simulink model "ES200A_CurrMeas"  (R2013b)
settings: Solver=FixedStepDiscrete  SolverMode=SingleTasking  StartTime=0.0  StopTime=1  FixedStep=0.000125  RelTol=1e-3
undefined symbols (not defined in the file): ARCHGLBPRM_2PI_ULS_F32, CurrMeasEolGainMax, CurrMeasEolGainMin, CurrMeasEolGainNrOfSample, CurrMeasEolGainNumer, CurrMeasEolMaxMotVel, CurrMeasEolOffsHiBrdgVltgMin, CurrMeasEolOffsHiCmuOffs, CurrMeasEolOffsLoCmuOffs, CurrMeasEolOffsMax, CurrMeasEolOffsMin, CurrMeasEolOffsNrOfSample, CurrMeasEolTranCntrThd, CurrMeasMinRqrdPhaOnTi, CurrMeasMotAgCompuDly, CurrMeasMotCurrAdcVlyWrmIninMax, CurrMeasMotCurrAdcVlyWrmIninMin, CurrMeasNtc0x05DFailStep, CurrMeasNtc0x05DPassStep, CurrMeasNtc0x06DFailStep, CurrMeasNtc0x06DPassStep, DEGREES30_MOTRAD_F32, DIFOFFSRNGCHKMAX_VOLT_F32, ELECGLBPRM_IVTRCNT_CNT_U08, ELECGLBPRM_STRTUPSTCURRMEASWRMININTESTSTRT_CNT_U08, FLTINJ_CURRMEAS_MOTCURRCORRDA, FLTINJ_CURRMEAS_MOTCURRCORRDD, FLTINJ_CURRMEAS_TESTOK, MAXCURRCORRD_AMPR_F32, PhaABCMeasdOutOfRng, PhaDEFMeasOutOfRng, SysGlbPrmMotPoleCnt
libraries: simulink x10, FixdToFloat x1
(part 4 of 7)

== system ES200A_CurrMeas/CurrMeas/CurrMeasInit1/If Action Subsystem1 ==
  Action Port : ActionPort  ActionType=else
  Constant{,1..5} (6 alike) : Constant  Value=0  OutDataTypeStr=single
  MotCurrOffsDeltaA : Outport
  MotCurrOffsDeltaB : Outport  Port=2
  MotCurrOffsDeltaC : Outport  Port=3
  MotCurrOffsDeltaD : Outport  Port=4
  MotCurrOffsDeltaE : Outport  Port=5
  MotCurrOffsDeltaF : Outport  Port=6
  wires:
  Constant2/1 -> MotCurrOffsDeltaC/1  "MotCurrOffDeltaC"
  Constant1/1 -> MotCurrOffsDeltaB/1  "MotCurrOffDeltaB"
  Constant/1 -> MotCurrOffsDeltaA/1  "MotCurrOffDeltaA"
  Constant3/1 -> MotCurrOffsDeltaD/1
  Constant4/1 -> MotCurrOffsDeltaE/1
  Constant5/1 -> MotCurrOffsDeltaF/1

== system ES200A_CurrMeas/CurrMeas/CurrMeasOffsReadReq/CopyRight2 ==

== system ES200A_CurrMeas/CurrMeas/CurrMeasOffsWrReq/CopyRight2 ==

== system ES200A_CurrMeas/CurrMeas/CurrMeasOffsWrReq/IF ==
  CurrMeasEolOffsHiBrdgVltg_ArgIn : Inport  RequirementInfo={} %GIDa_812a1a2f_8d9b_493f_8d38_cf559d2e2313  OutDataTypeStr=single
  CurrMeasMotCurrOffsDifA_ArgIn : Inport  RequirementInfo={} %GIDa_620df217_6d23_4379_b697_2438223fdb1e  Port=2  OutDataTypeStr=single
  CurrMeasMotCurrOffsLoAvrgA_ArgIn : Inport  RequirementInfo={} %GIDa_fbdbb2e3_d8ba_4172_b27f_3be627a5f176  Port=3  OutDataTypeStr=single
  CurrMeasMotCurrOffsLoAvrgB_ArgIn : Inport  RequirementInfo={} %GIDa_4342fbfc_d634_403b_9b29_d8803beea53e  Port=4  OutDataTypeStr=single
  CurrMeasMotCurrOffsLoAvrgC_ArgIn : Inport  RequirementInfo={} %GIDa_1155a904_daa1_442b_9b3a_76183cfeb8de  Port=5  OutDataTypeStr=single
  CurrMeasMotCurrOffsLoAvrgD_ArgIn : Inport  RequirementInfo={} %GIDa_b5928048_b518_475c_bd85_7d449910b834  Port=6  OutDataTypeStr=single
  CurrMeasMotCurrOffsLoAvrgE_ArgIn : Inport  RequirementInfo={} %GIDa_2f4f2a2a_6567_449e_882d_b458829ff196  Port=7  OutDataTypeStr=single
  CurrMeasMotCurrOffsLoAvrgF_ArgIn : Inport  RequirementInfo={} %GIDa_a7fe6648_99b2_41ba_8ec9_da3c20c2e7af  Port=8  OutDataTypeStr=single
  CurrMeasMotCurrOffsDifB_ArgIn : Inport  RequirementInfo={} %GIDa_17cf677d_9485_4eb6_bf0d_5d95365246ca  Port=9  OutDataTypeStr=single
  CurrMeasMotCurrOffsDifC_ArgIn : Inport  RequirementInfo={} %GIDa_8d171d0b_2ff9_462a_9ae6_84a29f9d80d8  Port=10  OutDataTypeStr=single
  CurrMeasMotCurrOffsDifD_ArgIn : Inport  RequirementInfo={} %GIDa_84414505_75c9_4dd9_ba80_d7374193ac56  Port=11  OutDataTypeStr=single
  CurrMeasMotCurrOffsDifE_ArgIn : Inport  RequirementInfo={} %GIDa_d54e2248_e490_46ca_9d40_ef0ba9a5a858  Port=12  OutDataTypeStr=single
  CurrMeasMotCurrOffsDifF_ArgIn : Inport  RequirementInfo={} %GIDa_15e5f242_fd24_4678_b9cf_ed0d82bfd499  Port=13  OutDataTypeStr=single
  Action Port : ActionPort  ActionType=then
  Constant14 : Constant  OutDataTypeStr=single
  CurrMeasEolOffsCalSet : DataStoreWrite  RequirementInfo={'linktype_rmi_doors' '000089bc (/ESG Group/FDD Module Requirements/EA4 Specific/ES200A_CurrMeas)' '#ES200A_280' 'true' 'REQ: ES200A_280' '' } %GIDa_65bd6eae_4bc4_46b4_a91f_58c4237add93  DataStoreName=CurrMeasEolOffsCalSet  DataStoreElements=CurrMeasEolOffsCalSet.CurrMeasEolOffsHiBrdgVltg#CurrMeasEolOffsCalSet.CurrMeasMotCurrEolOffsDifA#CurrMeasEolOffsCalSet.CurrMeasMotCurrEolOffsDifB#CurrMeasEolOffsCalSet.CurrMeasMotCurrEolOffsDifC#CurrMeasEolOffsCalSet.CurrMeasMotCurrEolOffsDifD#CurrMeasEolOffsCalSet.CurrMeasMotCurrEolOffsDifE#CurrMeasEolOffsCalSet.CurrMeasMotCurrEolOffsDifF#CurrMeasEolOffsCalSet.CurrMeasMotCurrOffsLoAvrgA#CurrMeasEolOffsCalSet.CurrMeasMotCurrOffsLoAvrgB#CurrMeasEolOffsCalSet.CurrMeasMotCurrOffsLoAvrgC#CurrMeasEolOffsCalSet.CurrMeasMotCurrOffsLoAvrgD#CurrMeasEolOffsCalSet.CurrMeasMotCurrOffsLoAvrgE#CurrMeasEolOffsCalSet.CurrMeasMotCurrOffsLoAvrgF
  CurrMeasEolOffsCalSet_SetRamBlockStatus : Subsystem  RequirementInfo={'linktype_rmi_doors' '000089bc (/ESG Group/FDD Module Requirements/EA4 Specific/ES200A_CurrMeas)' '#ES200A_280' 'true' 'REQ: ES200A_280' '' } %GIDa_fdbbe63c_7b7e_430e_a45c_f1a2eec3b0d3  TreatAsAtomicUnit=on
  Positive Response : Constant  Value=0
  CurrMeasOffsWrReqSts : Outport  RequirementInfo={} %GIDa_d6bd7840_4b1f_429e_aa0e_09addb50176a
  wires:
  CurrMeasMotCurrOffsDifB_ArgIn/1 -> CurrMeasEolOffsCalSet/3
  CurrMeasMotCurrOffsDifA_ArgIn/1 -> CurrMeasEolOffsCalSet/2
  CurrMeasMotCurrOffsLoAvrgC_ArgIn/1 -> CurrMeasEolOffsCalSet/10
  CurrMeasMotCurrOffsLoAvrgD_ArgIn/1 -> CurrMeasEolOffsCalSet/11
  CurrMeasMotCurrOffsLoAvrgF_ArgIn/1 -> CurrMeasEolOffsCalSet/13
  CurrMeasMotCurrOffsDifF_ArgIn/1 -> CurrMeasEolOffsCalSet/7
  CurrMeasMotCurrOffsDifC_ArgIn/1 -> CurrMeasEolOffsCalSet/4
  CurrMeasMotCurrOffsDifE_ArgIn/1 -> CurrMeasEolOffsCalSet/6
  CurrMeasMotCurrOffsLoAvrgB_ArgIn/1 -> CurrMeasEolOffsCalSet/9
  CurrMeasMotCurrOffsDifD_ArgIn/1 -> CurrMeasEolOffsCalSet/5
  CurrMeasMotCurrOffsLoAvrgA_ArgIn/1 -> CurrMeasEolOffsCalSet/8
  CurrMeasMotCurrOffsLoAvrgE_ArgIn/1 -> CurrMeasEolOffsCalSet/12
  Constant14/1 -> CurrMeasEolOffsCalSet_SetRamBlockStatus/1("BlockChanged ")
  CurrMeasEolOffsHiBrdgVltg_ArgIn/1 -> CurrMeasEolOffsCalSet/1
  Positive Response/1 -> CurrMeasOffsWrReqSts/1

== system ES200A_CurrMeas/CurrMeas/CurrMeasOffsWrReq/else  ==
  Action Port : ActionPort  ActionType=else
  Negative Response : Constant
  CurrMeasOffsWrReqSts : Outport  RequirementInfo={} %GIDa_bbade129_568d_4f6a_aeaa_1c5484c89fdb
  wires:
  Negative Response/1 -> CurrMeasOffsWrReqSts/1

== system ES200A_CurrMeas/CurrMeas/CurrMeasPer1/CopyRight2 ==

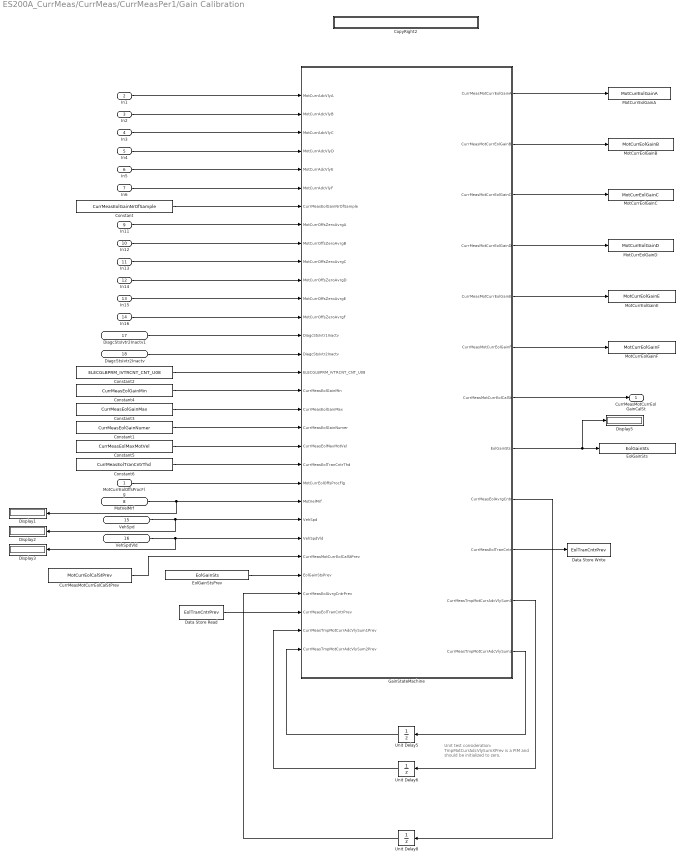
== system ES200A_CurrMeas/CurrMeas/CurrMeasPer1/Gain Calibration ==
  note: Unit test consideration:
      | TmpMotCurrAdcVlySumXPrev is a PIM
      | and should be initialized to zero.
  MotCurrEolOffsProcFlg : Inport
  In1 : Inport  Port=2
  In2 : Inport  Port=3
  In3 : Inport  Port=4
  In4 : Inport  Port=5
  In5 : Inport  Port=6
  In6 : Inport  Port=7
  MotVelMrf : Inport  RequirementInfo={} %GIDa_a7b78662_7cf0_48ed_9f87_08134d024c78  Port=8  OutDataTypeStr=single
  In11 : Inport  Port=9
  In12 : Inport  Port=10
  In13 : Inport  Port=11
  In14 : Inport  Port=12
  In15 : Inport  Port=13
  In16 : Inport  Port=14
  VehSpd : Inport  RequirementInfo={} %GIDa_c841d099_fc23_4afc_9dd2_bf4d1285ca82  Port=15
  VehSpdVld : Inport  RequirementInfo={} %GIDa_a5c49bc6_dd19_4849_b83d_4c3bf1157af9  Port=16  OutDataTypeStr=single
  DiagcStsIvtr2Inactv1 : Inport  RequirementInfo={} %GIDa_8700043e_90fa_4116_85b4_a3555476b354  Port=17
  DiagcStsIvtr2Inactv : Inport  RequirementInfo={} %GIDa_425966d8_d289_4e11_9dbb_57044454bfa8  Port=18
  Constant : Constant  Value=CurrMeasEolGainNrOfSample
  Constant1 : Constant  Value=CurrMeasEolGainNumer
  Constant2 : Constant  Value=ELECGLBPRM_IVTRCNT_CNT_U08  OutDataTypeStr=uint8
  Constant3 : Constant  Value=CurrMeasEolGainMax
  Constant4 : Constant  Value=CurrMeasEolGainMin
  Constant5 : Constant  Value=CurrMeasEolMaxMotVel
  Constant6 : Constant  Value=CurrMeasEolTranCntrThd
  CopyRight2 : Subsystem  Description=|  mask(Copyright Information){none=on}
      | Copyright info block.                                               
      |                                                                     
      | Place copyright information at the top of every subsystem in design.
      mask prompts: none "No parameters"
      mask help: Place copyright information at the top of every subsystem in design.
      mask Display:
      | NxtrConf = 'Nexteer Confidential';
      | 
      | sys = bdroot; %handle for the current model ("system")
      | first = get_param(sys,'Created');
      | first = first(end-3:end);  %year is last four digits
      | 
      | last = get_param(sys,'LastModifiedDate');
      | if isempty(last)
      |     last = datestr(now,'yyyy');
      | else
      |     last = last(end-3:end);
      | end
      | 
      | if strcmp(first,last)
      |     fprintf('%s -- Copyright %s Nexteer',NxtrConf,first)
      | else
      |     fprintf('%s -- %s%s- %s Nexteer',NxtrConf,char(169),first,last)
      | end
  CurrMeasMotCurrEolCalStPrev : DataStoreRead  DataStoreName=MotCurrEolCalStPrev  DataStoreElements=MotCurrEolCalStPrev
  Data Store Read : DataStoreRead  DataStoreName=EolTranCntrPrev
  Data Store Write : DataStoreWrite  DataStoreName=EolTranCntrPrev
  Display{1..3,5} (4 alike) : Display
  EolGainSts : DataStoreWrite  DataStoreName=EolGainSts
  EolGainStsPrev : DataStoreRead  DataStoreName=EolGainSts  DataStoreElements=EolGainSts
  GainStateMachine : Stateflow chart  RequirementInfo={'linktype_rmi_doors' '000089bc (/ESG Group/FDD Module Requirements/EA4 Specific/ES200A_CurrMeas)' '#ES200A_174' 'true' 'REQ: ES200A_174' '' } %GIDa_289e43b1_cfe4_41ba_9e49_3210dfe736ba  TreatAsAtomicUnit=on
  MotCurrEolGainA : DataStoreWrite  RequirementInfo={} %GIDa_13893fc7_c204_439f_bffc_cfe8ef3246c0  DataStoreName=MotCurrEolGainA
  MotCurrEolGainB : DataStoreWrite  RequirementInfo={} %GIDa_bd072951_11b3_473d_b14d_56675fe847ea  DataStoreName=MotCurrEolGainB
  MotCurrEolGainC : DataStoreWrite  RequirementInfo={} %GIDa_85f7aa39_8d03_4989_9937_397e0bbdc0c3  DataStoreName=MotCurrEolGainC
  MotCurrEolGainD : DataStoreWrite  RequirementInfo={} %GIDa_b5965ed2_4a8c_4234_8376_930d7494d8ae  DataStoreName=MotCurrEolGainD
  MotCurrEolGainE : DataStoreWrite  RequirementInfo={} %GIDa_5641d146_2eac_4d29_ad9c_8f8105bea573  DataStoreName=MotCurrEolGainE
  MotCurrEolGainF : DataStoreWrite  RequirementInfo={} %GIDa_25d2bb4a_a4ab_4b72_9cc3_33d4fd2a8c29  DataStoreName=MotCurrEolGainF
  Unit Delay5 : UnitDelay  SampleTime=-1  StateName=TmpMotCurrAdcVlySum2Prev  StateMustResolveToSignalObject=on
      settings: AttributesFormatString=|
      | State Variable:
      | %<StateName>
  Unit Delay6 : UnitDelay  SampleTime=-1  StateName=TmpMotCurrAdcVlySum1Prev  StateMustResolveToSignalObject=on
      settings: AttributesFormatString=|
      | State Variable:
      | %<StateName>
  Unit Delay8 : UnitDelay  SampleTime=-1  StateName=GainEolAvrgCntrPrev  StateMustResolveToSignalObject=on
      settings: AttributesFormatString=|
      | State Variable:
      | %<StateName>
  CurrMeasMotCurrEolGainCalSt : Outport  OutDataTypeStr=Enum: MotCurrEolCalSt2
  wires:
  GainStateMachine/1(CurrMeasMotCurrEolGainA) -> MotCurrEolGainA/1
  GainStateMachine/2(CurrMeasMotCurrEolGainB) -> MotCurrEolGainB/1
  GainStateMachine/3(CurrMeasMotCurrEolGainC) -> MotCurrEolGainC/1
  GainStateMachine/5(CurrMeasMotCurrEolGainE) -> MotCurrEolGainE/1
  GainStateMachine/6(CurrMeasMotCurrEolGainF) -> MotCurrEolGainF/1
  GainStateMachine/4(CurrMeasMotCurrEolGainD) -> MotCurrEolGainD/1
  GainStateMachine/8(EolGainSts) -> Display5/1, EolGainSts/1
  GainStateMachine/7(CurrMeasMotCurrEolCalSt) -> CurrMeasMotCurrEolGainCalSt/1
  In14/1 -> GainStateMachine/11(MotCurrOffsZeroAvrgD)
  In15/1 -> GainStateMachine/12(MotCurrOffsZeroAvrgE)
  In16/1 -> GainStateMachine/13(MotCurrOffsZeroAvrgF)
  In11/1 -> GainStateMachine/8(MotCurrOffsZeroAvrgA)
  In12/1 -> GainStateMachine/9(MotCurrOffsZeroAvrgB)
  In13/1 -> GainStateMachine/10(MotCurrOffsZeroAvrgC)
  Constant5/1 -> GainStateMachine/20(CurrMeasEolMaxMotVel)
  Constant6/1 -> GainStateMachine/21(CurrMeasEolTranCntrThd)
  Constant3/1 -> GainStateMachine/18(CurrMeasEolGainMax)
  Constant1/1 -> GainStateMachine/19(CurrMeasEolGainNumer)
  Constant4/1 -> GainStateMachine/17(CurrMeasEolGainMin)
  MotVelMrf/1 -> Display1/1, GainStateMachine/23(MotVelMrf)
  EolGainStsPrev/1 -> GainStateMachine/27(EolGainStsPrev)
  VehSpdVld/1 -> Display3/1, GainStateMachine/25(VehSpdVld)
  VehSpd/1 -> Display2/1, GainStateMachine/24(VehSpd)
  CurrMeasMotCurrEolCalStPrev/1 -> GainStateMachine/26(CurrMeasMotCurrEolCalStPrev)
  MotCurrEolOffsProcFlg/1 -> GainStateMachine/22(MotCurrEolOffsProcFlg)
  GainStateMachine/9(CurrMeasEolAvrgCntr) -> Unit Delay8/1
  Unit Delay8/1 -> GainStateMachine/28(CurrMeasEolAvrgCntrPrev)
  GainStateMachine/11(CurrMeasTmpMotCurrAdcVlySum1) -> Unit Delay6/1
  Unit Delay6/1 -> GainStateMachine/30(CurrMeasTmpMotCurrAdcVlySum1Prev)
  GainStateMachine/12(CurrMeasTmpMotCurrAdcVlySum2) -> Unit Delay5/1
  Unit Delay5/1 -> GainStateMachine/31(CurrMeasTmpMotCurrAdcVlySum2Prev)
  Constant/1 -> GainStateMachine/7(CurrMeasEolGainNrOfSample)
  In4/1 -> GainStateMachine/4(MotCurrAdcVlyD)
  In3/1 -> GainStateMachine/3(MotCurrAdcVlyC)
  In1/1 -> GainStateMachine/1(MotCurrAdcVlyA)
  In6/1 -> GainStateMachine/6(MotCurrAdcVlyF)
  In5/1 -> GainStateMachine/5(MotCurrAdcVlyE)
  In2/1 -> GainStateMachine/2(MotCurrAdcVlyB)
  Constant2/1 -> GainStateMachine/16(ELECGLBPRM_IVTRCNT_CNT_U08)
  DiagcStsIvtr2Inactv1/1 -> GainStateMachine/14(DiagcStsIvtr1Inactv)
  DiagcStsIvtr2Inactv/1 -> GainStateMachine/15(DiagcStsIvtr2Inactv)
  GainStateMachine/10(CurrMeasEolTranCntr) -> Data Store Write/1
  Data Store Read/1 -> GainStateMachine/29(CurrMeasEolTranCntrPrev)

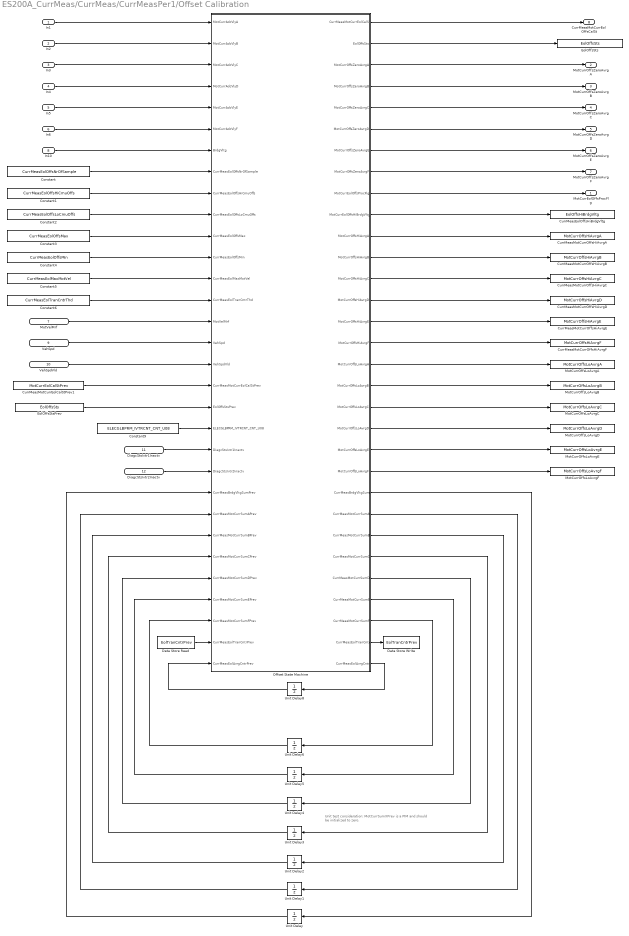
== system ES200A_CurrMeas/CurrMeas/CurrMeasPer1/Offset Calibration ==
  note: Unit test consideration:
      | MotCurrSumXPrev is a PIM and should be initialized to zero.
  In1 : Inport
  In2 : Inport  Port=2
  In3 : Inport  Port=3
  In4 : Inport  Port=4
  In5 : Inport  Port=5
  In6 : Inport  Port=6
  MotVelMrf : Inport  RequirementInfo={} %GIDa_78f9eb59_5144_46af_979c_575c98288e43  Port=7  OutDataTypeStr=single
  In10 : Inport  Port=8
  VehSpd : Inport  RequirementInfo={} %GIDa_7dd3d444_7490_4948_b310_12c64a4e793e  Port=9
  VehSpdVld : Inport  RequirementInfo={} %GIDa_8fb497df_f50d_4138_b2fb_eb56850af411  Port=10
  DiagcStsIvtr1Inactv : Inport  RequirementInfo={} %GIDa_e6a44153_6521_4486_9f01_84c87aee9f80  Port=11
  DiagcStsIvtr2Inactv : Inport  RequirementInfo={} %GIDa_b941d451_ac68_4839_91af_6c254399bdf9  Port=12
  Constant : Constant  Value=CurrMeasEolOffsNrOfSample
  Constant1 : Constant  Value=CurrMeasEolOffsHiCmuOffs
  Constant2 : Constant  Value=CurrMeasEolOffsLoCmuOffs
  Constant3 : Constant  Value=CurrMeasEolOffsMax
  Constant4 : Constant  Value=CurrMeasEolOffsMin
  Constant5 : Constant  Value=CurrMeasEolMaxMotVel
  Constant6 : Constant  Value=CurrMeasEolTranCntrThd
  Constant9 : Constant  Value=ELECGLBPRM_IVTRCNT_CNT_U08  OutDataTypeStr=uint8
  CurrMeasEolOffsHiBrdgVltg : DataStoreWrite  RequirementInfo={} %GIDa_f0dd7216_1c54_4df2_acb2_47771392ab80  DataStoreName=EolOffsHiBrdgVltg  DataStoreElements=EolOffsHiBrdgVltg
  CurrMeasMotCurrEolCalStPrev1 : DataStoreRead  DataStoreName=MotCurrEolCalStPrev  DataStoreElements=MotCurrEolCalStPrev
  CurrMeasMotCurrOffsHiAvrgA : DataStoreWrite  DataStoreName=MotCurrOffsHiAvrgA  DataStoreElements=MotCurrOffsHiAvrgA
  CurrMeasMotCurrOffsHiAvrgB : DataStoreWrite  DataStoreName=MotCurrOffsHiAvrgB  DataStoreElements=MotCurrOffsHiAvrgB
  CurrMeasMotCurrOffsHiAvrgC : DataStoreWrite  DataStoreName=MotCurrOffsHiAvrgC  DataStoreElements=MotCurrOffsHiAvrgC
  CurrMeasMotCurrOffsHiAvrgD : DataStoreWrite  DataStoreName=MotCurrOffsHiAvrgD  DataStoreElements=MotCurrOffsHiAvrgD
  CurrMeasMotCurrOffsHiAvrgE : DataStoreWrite  DataStoreName=MotCurrOffsHiAvrgE  DataStoreElements=MotCurrOffsHiAvrgE
  CurrMeasMotCurrOffsHiAvrgF : DataStoreWrite  DataStoreName=MotCurrOffsHiAvrgF  DataStoreElements=MotCurrOffsHiAvrgF
  Data Store Read : DataStoreRead  DataStoreName=EolTranCntrPrev
  Data Store Write : DataStoreWrite  DataStoreName=EolTranCntrPrev
  EolOffsSts : DataStoreWrite  DataStoreName=EolOffsSts  DataStoreElements=EolOffsSts
  EolOffsStsPrev : DataStoreRead  DataStoreName=EolOffsSts  DataStoreElements=EolOffsSts
  MotCurrOffsLoAvrgA : DataStoreWrite  RequirementInfo={} %GIDa_67dd0541_ce70_473f_aba6_79f393300d3a  DataStoreName=MotCurrOffsLoAvrgA  DataStoreElements=MotCurrOffsLoAvrgA
  MotCurrOffsLoAvrgB : DataStoreWrite  RequirementInfo={} %GIDa_b1bf0627_1797_446c_b82a_a08e5020abc1  DataStoreName=MotCurrOffsLoAvrgB  DataStoreElements=MotCurrOffsLoAvrgB
  MotCurrOffsLoAvrgC : DataStoreWrite  RequirementInfo={} %GIDa_6853784a_55cf_4a5e_9507_3e15451cdc3f  DataStoreName=MotCurrOffsLoAvrgC  DataStoreElements=MotCurrOffsLoAvrgC
  MotCurrOffsLoAvrgD : DataStoreWrite  RequirementInfo={} %GIDa_5af9b3b8_7792_41d4_b90d_39024460e08e  DataStoreName=MotCurrOffsLoAvrgD  DataStoreElements=MotCurrOffsLoAvrgD
  MotCurrOffsLoAvrgE : DataStoreWrite  RequirementInfo={} %GIDa_cce00581_4c40_4f0f_85ad_eed2dba881f4  DataStoreName=MotCurrOffsLoAvrgE  DataStoreElements=MotCurrOffsLoAvrgE
  MotCurrOffsLoAvrgF : DataStoreWrite  RequirementInfo={} %GIDa_2835df82_1ac0_4777_a205_58cb6597b789  DataStoreName=MotCurrOffsLoAvrgF  DataStoreElements=MotCurrOffsLoAvrgF
  Offset State Machine : Stateflow chart  RequirementInfo={'linktype_rmi_doors' '000089bc (/ESG Group/FDD Module Requirements/EA4 Specific/ES200A_CurrMeas)' '#ES200A_135' 'true' 'REQ: ES200A_135' '' } %GIDa_67714aa5_9ea9_405b_a1a2_441ce02afd28  TreatAsAtomicUnit=on
  Unit Delay : UnitDelay  SampleTime=-1  StateName=BrdgVltgSumPrev  StateMustResolveToSignalObject=on
      settings: AttributesFormatString=|
      | State Variable:
      | %<StateName>
  Unit Delay1 : UnitDelay  SampleTime=-1  StateName=MotCurrSumAPrev  StateMustResolveToSignalObject=on
      settings: AttributesFormatString=|
      | State Variable:
      | %<StateName>
  Unit Delay2 : UnitDelay  SampleTime=-1  StateName=MotCurrSumBPrev  StateMustResolveToSignalObject=on
      settings: AttributesFormatString=|
      | State Variable:
      | %<StateName>
  Unit Delay3 : UnitDelay  SampleTime=-1  StateName=MotCurrSumCPrev  StateMustResolveToSignalObject=on
      settings: AttributesFormatString=|
      | State Variable:
      | %<StateName>
  Unit Delay4 : UnitDelay  SampleTime=-1  StateName=MotCurrSumDPrev  StateMustResolveToSignalObject=on
      settings: AttributesFormatString=|
      | State Variable:
      | %<StateName>
  Unit Delay5 : UnitDelay  SampleTime=-1  StateName=MotCurrSumEPrev  StateMustResolveToSignalObject=on
      settings: AttributesFormatString=|
      | State Variable:
      | %<StateName>
  Unit Delay6 : UnitDelay  SampleTime=-1  StateName=MotCurrSumFPrev  StateMustResolveToSignalObject=on
      settings: AttributesFormatString=|
      | State Variable:
      | %<StateName>
  Unit Delay8 : UnitDelay  SampleTime=-1  StateName=OffsEolAvrgCntrPrev  StateMustResolveToSignalObject=on
      settings: AttributesFormatString=|
      | State Variable:
      | %<StateName>
  "MotCurrEolOffsProcFlg " : Outport
  MotCurrOffsZeroAvrgA : Outport  Port=2
  MotCurrOffsZeroAvrgB : Outport  Port=3
  MotCurrOffsZeroAvrgC : Outport  Port=4
  MotCurrOffsZeroAvrgD : Outport  Port=5
  MotCurrOffsZeroAvrgE : Outport  Port=6
  MotCurrOffsZeroAvrgF : Outport  Port=7
  CurrMeasMotCurrEolOffsCalSt : Outport  Port=8  OutDataTypeStr=Enum: MotCurrEolCalSt2
  wires:
  In1/1 -> Offset State Machine/1(MotCurrAdcVlyA)
  In2/1 -> Offset State Machine/2(MotCurrAdcVlyB)
  In3/1 -> Offset State Machine/3(MotCurrAdcVlyC)
  In10/1 -> Offset State Machine/7(BrdgVltg)
  Constant1/1 -> Offset State Machine/9(CurrMeasEolOffsHiCmuOffs)
  Constant2/1 -> Offset State Machine/10(CurrMeasEolOffsLoCmuOffs)
  Constant/1 -> Offset State Machine/8(CurrMeasEolOffsNrOfSample)
  In6/1 -> Offset State Machine/6(MotCurrAdcVlyF)
  In5/1 -> Offset State Machine/5(MotCurrAdcVlyE)
  In4/1 -> Offset State Machine/4(MotCurrAdcVlyD)
  Constant3/1 -> Offset State Machine/11(CurrMeasEolOffsMax)
  Constant4/1 -> Offset State Machine/12(CurrMeasEolOffsMin)
  Constant5/1 -> Offset State Machine/13(CurrMeasEolMaxMotVel)
  Constant6/1 -> Offset State Machine/14(CurrMeasEolTranCntrThd)
  MotVelMrf/1 -> Offset State Machine/15(MotVelMrf)
  VehSpd/1 -> Offset State Machine/16(VehSpd)
  VehSpdVld/1 -> Offset State Machine/17(VehSpdVld)
  Offset State Machine/3(MotCurrOffsZeroAvrgA) -> MotCurrOffsZeroAvrgA/1
  Offset State Machine/4(MotCurrOffsZeroAvrgB) -> MotCurrOffsZeroAvrgB/1
  Offset State Machine/5(MotCurrOffsZeroAvrgC) -> MotCurrOffsZeroAvrgC/1
  Offset State Machine/6(MotCurrOffsZeroAvrgD) -> MotCurrOffsZeroAvrgD/1
  Offset State Machine/7(MotCurrOffsZeroAvrgE) -> MotCurrOffsZeroAvrgE/1
  Offset State Machine/8(MotCurrOffsZeroAvrgF) -> MotCurrOffsZeroAvrgF/1
  CurrMeasMotCurrEolCalStPrev1/1 -> Offset State Machine/18(CurrMeasMotCurrEolCalStPrev)
  Offset State Machine/9(MotCurrEolOffsProcFlg) -> "MotCurrEolOffsProcFlg "/1
  Offset State Machine/2(EolOffsSts) -> EolOffsSts/1
  EolOffsStsPrev/1 -> Offset State Machine/19(EolOffsStsPrev)
  Offset State Machine/1(CurrMeasMotCurrEolCalSt) -> CurrMeasMotCurrEolOffsCalSt/1
  Offset State Machine/23(CurrMeasBrdgVltgSum) -> Unit Delay/1
  Unit Delay/1 -> Offset State Machine/23(CurrMeasBrdgVltgSumPrev)
  Offset State Machine/24(CurrMeasMotCurrSumA) -> Unit Delay1/1
  Offset State Machine/25(CurrMeasMotCurrSumB) -> Unit Delay2/1
  Offset State Machine/26(CurrMeasMotCurrSumC) -> Unit Delay3/1
  Offset State Machine/27(CurrMeasMotCurrSumD) -> Unit Delay4/1
  Offset State Machine/28(CurrMeasMotCurrSumE) -> Unit Delay5/1
  Offset State Machine/29(CurrMeasMotCurrSumF) -> Unit Delay6/1
  Offset State Machine/31(CurrMeasEolAvrgCntr) -> Unit Delay8/1
  Unit Delay1/1 -> Offset State Machine/24(CurrMeasMotCurrSumAPrev)
  Unit Delay2/1 -> Offset State Machine/25(CurrMeasMotCurrSumBPrev)
  Unit Delay3/1 -> Offset State Machine/26(CurrMeasMotCurrSumCPrev)
  Unit Delay4/1 -> Offset State Machine/27(CurrMeasMotCurrSumDPrev)
  Unit Delay5/1 -> Offset State Machine/28(CurrMeasMotCurrSumEPrev)
  Unit Delay6/1 -> Offset State Machine/29(CurrMeasMotCurrSumFPrev)
  Unit Delay8/1 -> Offset State Machine/31(CurrMeasEolAvrgCntrPrev)
  Offset State Machine/17(MotCurrOffsLoAvrgA) -> MotCurrOffsLoAvrgA/1
  Offset State Machine/18(MotCurrOffsLoAvrgB) -> MotCurrOffsLoAvrgB/1
  Offset State Machine/19(MotCurrOffsLoAvrgC) -> MotCurrOffsLoAvrgC/1
  Offset State Machine/20(MotCurrOffsLoAvrgD) -> MotCurrOffsLoAvrgD/1
  Offset State Machine/21(MotCurrOffsLoAvrgE) -> MotCurrOffsLoAvrgE/1
  Offset State Machine/22(MotCurrOffsLoAvrgF) -> MotCurrOffsLoAvrgF/1
  Offset State Machine/11(MotCurrOffsHiAvrgA) -> CurrMeasMotCurrOffsHiAvrgA/1
  Offset State Machine/12(MotCurrOffsHiAvrgB) -> CurrMeasMotCurrOffsHiAvrgB/1
  Offset State Machine/13(MotCurrOffsHiAvrgC) -> CurrMeasMotCurrOffsHiAvrgC/1
  Offset State Machine/14(MotCurrOffsHiAvrgD) -> CurrMeasMotCurrOffsHiAvrgD/1
  Offset State Machine/15(MotCurrOffsHiAvrgE) -> CurrMeasMotCurrOffsHiAvrgE/1
  Offset State Machine/16(MotCurrOffsHiAvrgF) -> CurrMeasMotCurrOffsHiAvrgF/1
  Constant9/1 -> Offset State Machine/20(ELECGLBPRM_IVTRCNT_CNT_U08)
  DiagcStsIvtr2Inactv/1 -> Offset State Machine/22(DiagcStsIvtr2Inactv)
  DiagcStsIvtr1Inactv/1 -> Offset State Machine/21(DiagcStsIvtr1Inactv)
  Offset State Machine/10(MotCurrEolOffsHiBrdgVltg) -> CurrMeasEolOffsHiBrdgVltg/1
  Data Store Read/1 -> Offset State Machine/30(CurrMeasEolTranCntrPrev)
  Offset State Machine/30(CurrMeasEolTranCntr) -> Data Store Write/1

== system ES200A_CurrMeas/CurrMeas/CurrMeasPer2/Chart1/CalcMotCurrMotAgCorrd ==
  note: [RADIAN]
  note: Converting from Cnt to Rev
  note: [RADIAN]
  note: [RADIAN]
  note: [RADIAN]
  note: [Cnts]
  note: [Rev]
  MotCtrlMotAgElec : Inport
  MotCtrlMotElecMeclPolarity : Inport  Port=2
  MotCtrlMotVelMrf : Inport  Port=3
  CurrMeasMotAgCompuDly : Inport  Port=4
  f : TriggerPort  TriggerType=function-call
      settings: CopyFcn=Stateflow.SLINSF.SimulinkMan.removeBlockPreDeleteFcn  PreDeleteFcn=Stateflow.SLINSF.SimulinkMan.unsafePredeleteFcn
  +/- 2*Pi Rollover : Subsystem
  Add : Sum  Inputs=+-+
  Constant : Constant  Value=ARCHGLBPRM_2PI_ULS_F32  OutDataTypeStr=Inherit: Inherit via back propagation
  Constant1 : Constant  Value=DEGREES30_MOTRAD_F32
  Constant2 : Constant  Value=2  OutDataTypeStr=single
  Constant3 : Constant  Value=SysGlbPrmMotPoleCnt  OutDataTypeStr=single
  CopyRight2 : Subsystem  Description=|  mask(Copyright Information){none=on}
      | Copyright info block.                                               
      |                                                                     
      | Place copyright information at the top of every subsystem in design.
      mask prompts: none "No parameters"
      mask help: Place copyright information at the top of every subsystem in design.
      mask Display:
      | NxtrConf = 'Nexteer Confidential';
      | 
      | sys = bdroot; %handle for the current model ("system")
      | first = get_param(sys,'Created');
      | first = first(end-3:end);  %year is last four digits
      | 
      | last = get_param(sys,'LastModifiedDate');
      | if isempty(last)
      |     last = datestr(now,'yyyy');
      | else
      |     last = last(end-3:end);
      | end
      | 
      | if strcmp(first,last)
      |     fprintf('%s -- Copyright %s Nexteer',NxtrConf,first)
      | else
      |     fprintf('%s -- %s%s- %s Nexteer',NxtrConf,char(169),first,last)
      | end
  Divide : Product  Inputs=***
  Divide1 : Product  Inputs=**
  Divide2 : Product  Inputs=**
  Divide3 : Product  Inputs=*/
  FixdToFloat_f32_u16 (multiplying with 2E-16) : FixdToFloat/FixdToFloat_f32_u16  Param1=16
  Gain : Gain  Gain=1/1E9
  MotCtrlCurrMeasMotAgCorrd : Outport
  wires:
  MotCtrlMotVelMrf/1 -> Divide/2
  CurrMeasMotAgCompuDly/1 -> Gain/1
  MotCtrlMotAgElec/1 -> FixdToFloat_f32_u16 (multiplying with 2E-16)/1
  Constant/1 -> Divide1/2
  Divide1/1 -> Add/1  "MotAgCorrdElecRad"
  Divide/1 -> Add/3  "MotCurrMotAgDlyCmpRad"
  Gain/1 -> Divide/3
  Constant1/1 -> Divide2/1
  MotCtrlMotElecMeclPolarity/1 -> Divide2/2
  Divide2/1 -> Add/2  "Rad"
  Constant3/1 -> Divide3/1
  Constant2/1 -> Divide3/2
  Divide3/1 -> Divide/1
  FixdToFloat_f32_u16 (multiplying with 2E-16)/1 -> Divide1/1
  Add/1 -> +/- 2*Pi Rollover/1(MotAgCorrdRaw)
  +/- 2*Pi Rollover/1(MotCtrlCurrMeasMotAgCorrd) -> MotCtrlCurrMeasMotAgCorrd/1

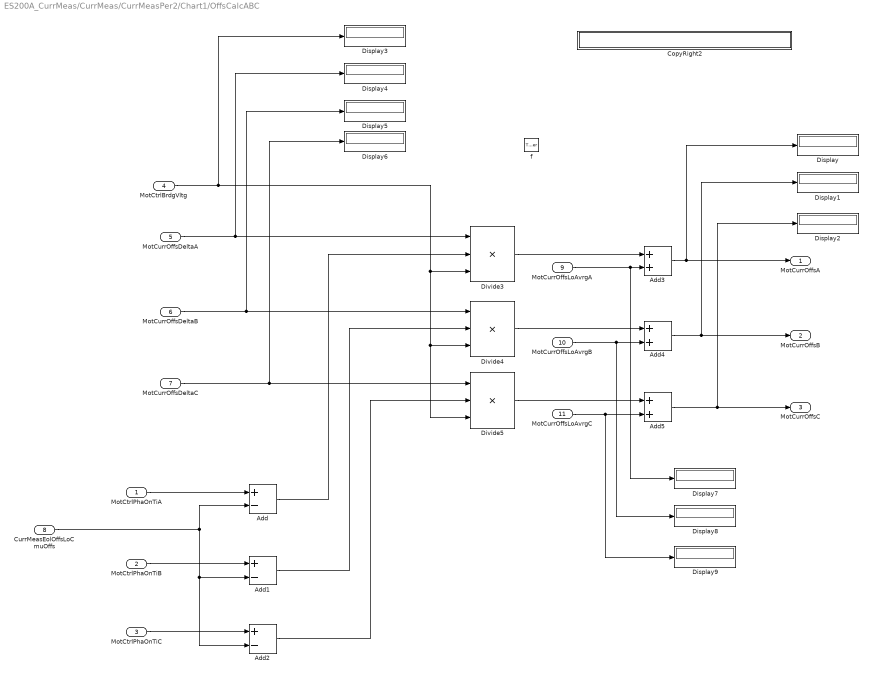
== system ES200A_CurrMeas/CurrMeas/CurrMeasPer2/Chart1/OffsCalcABC ==
  MotCtrlPhaOnTiA : Inport
  MotCtrlPhaOnTiB : Inport  Port=2
  MotCtrlPhaOnTiC : Inport  Port=3
  MotCtrlBrdgVltg : Inport  Port=4
  MotCurrOffsDeltaA : Inport  Port=5
  MotCurrOffsDeltaB : Inport  Port=6
  MotCurrOffsDeltaC : Inport  Port=7
  CurrMeasEolOffsLoCmuOffs : Inport  Port=8
  MotCurrOffsLoAvrgA : Inport  Port=9
  MotCurrOffsLoAvrgB : Inport  Port=10
  MotCurrOffsLoAvrgC : Inport  Port=11
  f : TriggerPort  TriggerType=function-call
      settings: CopyFcn=Stateflow.SLINSF.SimulinkMan.removeBlockPreDeleteFcn  PreDeleteFcn=Stateflow.SLINSF.SimulinkMan.unsafePredeleteFcn
  Add : Sum  Inputs=+-
  Add1 : Sum  Inputs=+-
  Add2 : Sum  Inputs=+-
  Add3 : Sum
  Add4 : Sum
  Add5 : Sum
  CopyRight2 : Subsystem  Description=|  mask(Copyright Information){none=on}
      | Copyright info block.                                               
      |                                                                     
      | Place copyright information at the top of every subsystem in design.
      mask prompts: none "No parameters"
      mask help: Place copyright information at the top of every subsystem in design.
      mask Display:
      | NxtrConf = 'Nexteer Confidential';
      | 
      | sys = bdroot; %handle for the current model ("system")
      | first = get_param(sys,'Created');
      | first = first(end-3:end);  %year is last four digits
      | 
      | last = get_param(sys,'LastModifiedDate');
      | if isempty(last)
      |     last = datestr(now,'yyyy');
      | else
      |     last = last(end-3:end);
      | end
      | 
      | if strcmp(first,last)
      |     fprintf('%s -- Copyright %s Nexteer',NxtrConf,first)
      | else
      |     fprintf('%s -- %s%s- %s Nexteer',NxtrConf,char(169),first,last)
      | end
  Display{,1..9} (10 alike) : Display
  Divide3 : Product  Inputs=***
  Divide4 : Product  Inputs=***
  Divide5 : Product  Inputs=***
  MotCurrOffsA : Outport
  MotCurrOffsB : Outport  Port=2
  MotCurrOffsC : Outport  Port=3
  wires:
  MotCtrlPhaOnTiA/1 -> Add/1
  MotCtrlPhaOnTiB/1 -> Add1/1
  MotCtrlPhaOnTiC/1 -> Add2/1
  CurrMeasEolOffsLoCmuOffs/1 -> Add2/2, Add1/2, Add/2
  Add/1 -> Divide3/2
  Add1/1 -> Divide4/2
  Add2/1 -> Divide5/2
  Divide3/1 -> Add3/1
  Divide4/1 -> Add4/1
  Divide5/1 -> Add5/1
  MotCurrOffsLoAvrgA/1 -> Display7/1, Add3/2
  MotCurrOffsLoAvrgB/1 -> Display8/1, Add4/2
  MotCurrOffsLoAvrgC/1 -> Display9/1, Add5/2
  Add3/1 -> Display/1, MotCurrOffsA/1
  Add4/1 -> Display1/1, MotCurrOffsB/1
  Add5/1 -> MotCurrOffsC/1, Display2/1
  MotCurrOffsDeltaA/1 -> Display4/1, Divide3/1
  MotCurrOffsDeltaB/1 -> Display5/1, Divide4/1
  MotCurrOffsDeltaC/1 -> Display6/1, Divide5/1
  MotCtrlBrdgVltg/1 -> Display3/1, Divide4/3, Divide5/3, Divide3/3

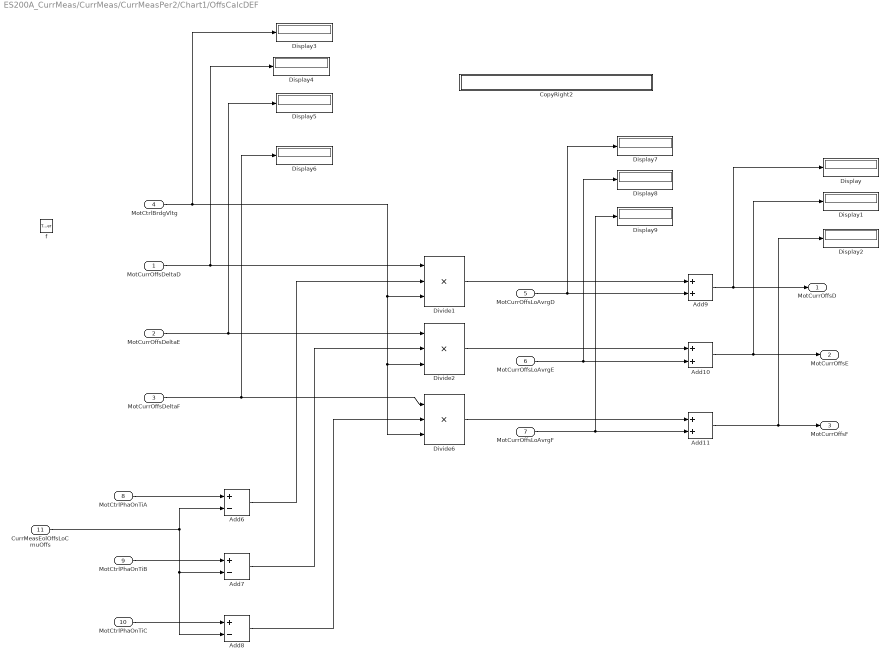
== system ES200A_CurrMeas/CurrMeas/CurrMeasPer2/Chart1/OffsCalcDEF ==
  MotCurrOffsDeltaD : Inport
  MotCurrOffsDeltaE : Inport  Port=2
  MotCurrOffsDeltaF : Inport  Port=3
  MotCtrlBrdgVltg : Inport  Port=4
  MotCurrOffsLoAvrgD : Inport  Port=5
  MotCurrOffsLoAvrgE : Inport  Port=6
  MotCurrOffsLoAvrgF : Inport  Port=7
  MotCtrlPhaOnTiA : Inport  Port=8
  MotCtrlPhaOnTiB : Inport  Port=9
  MotCtrlPhaOnTiC : Inport  Port=10
  CurrMeasEolOffsLoCmuOffs : Inport  Port=11
  f : TriggerPort  TriggerType=function-call
      settings: CopyFcn=Stateflow.SLINSF.SimulinkMan.removeBlockPreDeleteFcn  PreDeleteFcn=Stateflow.SLINSF.SimulinkMan.unsafePredeleteFcn
  Add10 : Sum
  Add11 : Sum
  Add6 : Sum  Inputs=+-
  Add7 : Sum  Inputs=+-
  Add8 : Sum  Inputs=+-
  Add9 : Sum
  CopyRight2 : Subsystem  Description=|  mask(Copyright Information){none=on}
      | Copyright info block.                                               
      |                                                                     
      | Place copyright information at the top of every subsystem in design.
      mask prompts: none "No parameters"
      mask help: Place copyright information at the top of every subsystem in design.
      mask Display:
      | NxtrConf = 'Nexteer Confidential';
      | 
      | sys = bdroot; %handle for the current model ("system")
      | first = get_param(sys,'Created');
      | first = first(end-3:end);  %year is last four digits
      | 
      | last = get_param(sys,'LastModifiedDate');
      | if isempty(last)
      |     last = datestr(now,'yyyy');
      | else
      |     last = last(end-3:end);
      | end
      | 
      | if strcmp(first,last)
      |     fprintf('%s -- Copyright %s Nexteer',NxtrConf,first)
      | else
      |     fprintf('%s -- %s%s- %s Nexteer',NxtrConf,char(169),first,last)
      | end
  Display{,1..9} (10 alike) : Display
  Divide1 : Product  Inputs=***
  Divide2 : Product  Inputs=***
  Divide6 : Product  Inputs=***
  MotCurrOffsD : Outport
  MotCurrOffsE : Outport  Port=2
  MotCurrOffsF : Outport  Port=3
  wires:
  MotCtrlPhaOnTiA/1 -> Add6/1
  MotCtrlPhaOnTiB/1 -> Add7/1
  MotCtrlPhaOnTiC/1 -> Add8/1
  CurrMeasEolOffsLoCmuOffs/1 -> Add8/2, Add7/2, Add6/2
  Add6/1 -> Divide1/2
  Add7/1 -> Divide2/2
  Add8/1 -> Divide6/2
  MotCtrlBrdgVltg/1 -> Display3/1, Divide2/3, Divide6/3, Divide1/3
  Divide1/1 -> Add9/1
  Divide2/1 -> Add10/1
  Divide6/1 -> Add11/1
  MotCurrOffsLoAvrgD/1 -> Display7/1, Add9/2
  MotCurrOffsLoAvrgE/1 -> Display8/1, Add10/2
  MotCurrOffsLoAvrgF/1 -> Display9/1, Add11/2
  Add9/1 -> Display/1, MotCurrOffsD/1
  Add10/1 -> Display1/1, MotCurrOffsE/1
  Add11/1 -> Display2/1, MotCurrOffsF/1
  MotCurrOffsDeltaD/1 -> Display4/1, Divide1/1
  MotCurrOffsDeltaE/1 -> Display5/1, Divide2/1
  MotCurrOffsDeltaF/1 -> Display6/1, Divide6/1

== system ES200A_CurrMeas/CurrMeas/CurrMeasPer2/Chart1/ProtocolChkENABC ==
  MotCtrlMotCurrAdcVlyAAdcFaild : Inport
  MotCtrlMotCurrAdcVlyBAdcFaild : Inport  Port=2
  MotCtrlMotCurrAdcVlyCAdcFaild : Inport  Port=3
  f : TriggerPort  TriggerType=function-call
      settings: CopyFcn=Stateflow.SLINSF.SimulinkMan.removeBlockPreDeleteFcn  PreDeleteFcn=Stateflow.SLINSF.SimulinkMan.unsafePredeleteFcn
  CopyRight2 : Subsystem  Description=|  mask(Copyright Information){none=on}
      | Copyright info block.                                               
      |                                                                     
      | Place copyright information at the top of every subsystem in design.
      mask prompts: none "No parameters"
      mask help: Place copyright information at the top of every subsystem in design.
      mask Display:
      | NxtrConf = 'Nexteer Confidential';
      | 
      | sys = bdroot; %handle for the current model ("system")
      | first = get_param(sys,'Created');
      | first = first(end-3:end);  %year is last four digits
      | 
      | last = get_param(sys,'LastModifiedDate');
      | if isempty(last)
      |     last = datestr(now,'yyyy');
      | else
      |     last = last(end-3:end);
      | end
      | 
      | if strcmp(first,last)
      |     fprintf('%s -- Copyright %s Nexteer',NxtrConf,first)
      | else
      |     fprintf('%s -- %s%s- %s Nexteer',NxtrConf,char(169),first,last)
      | end
  Display : Display
  Display1 : Display
  FLTINJ_CURRMEAS_MOTCURRCORRDA1 : Constant  Value=FLTINJ_CURRMEAS_TESTOK
  FltInj_u08 : Subsystem  RequirementInfo={'linktype_rmi_doors' '000089bc (/ESG Group/FDD Module Requirements/EA4 Specific/ES200A_CurrMeas)' '#ES200A_270' 'true' 'REQ: ES200A_270' '' } %GIDa_c3f30c2f_52ad_4d52_84d2_62824c43486f  TreatAsAtomicUnit=on  VariantControl=FltInj_sim  mask(Fault_Injection){}
      mask help: Fault Injection is a simulation only block for EA3 programs.
  Logical Operator : Logic  Operator=OR  Inputs=3  AllPortsSameDT=off  OutDataTypeStr=boolean
  Logical Operator1 : Logic  Operator=NOT  IconShape=distinctive  AllPortsSameDT=off  OutDataTypeStr=boolean
  PrtclChkENABC : Outport
  wires:
  FltInj_u08/1(Signal_Out) -> Display1/1, PrtclChkENABC/1
  FLTINJ_CURRMEAS_MOTCURRCORRDA1/1 -> FltInj_u08/2(Constant)
  MotCtrlMotCurrAdcVlyAAdcFaild/1 -> Logical Operator/1
  MotCtrlMotCurrAdcVlyBAdcFaild/1 -> Logical Operator/2
  MotCtrlMotCurrAdcVlyCAdcFaild/1 -> Logical Operator/3
  Logical Operator1/1 -> Display/1, FltInj_u08/1(Signal_In)
  Logical Operator/1 -> Logical Operator1/1

== system ES200A_CurrMeas/CurrMeas/CurrMeasPer2/Chart1/ProtocolChkENDEF ==
  MotCtrlMotCurrAdcVlyDAdcFaild : Inport
  MotCtrlMotCurrAdcVlyEAdcFaild : Inport  Port=2
  MotCtrlMotCurrAdcVlyFAdcFaild : Inport  Port=3
  f : TriggerPort  TriggerType=function-call
      settings: CopyFcn=Stateflow.SLINSF.SimulinkMan.removeBlockPreDeleteFcn  PreDeleteFcn=Stateflow.SLINSF.SimulinkMan.unsafePredeleteFcn
  CopyRight2 : Subsystem  Description=|  mask(Copyright Information){none=on}
      | Copyright info block.                                               
      |                                                                     
      | Place copyright information at the top of every subsystem in design.
      mask prompts: none "No parameters"
      mask help: Place copyright information at the top of every subsystem in design.
      mask Display:
      | NxtrConf = 'Nexteer Confidential';
      | 
      | sys = bdroot; %handle for the current model ("system")
      | first = get_param(sys,'Created');
      | first = first(end-3:end);  %year is last four digits
      | 
      | last = get_param(sys,'LastModifiedDate');
      | if isempty(last)
      |     last = datestr(now,'yyyy');
      | else
      |     last = last(end-3:end);
      | end
      | 
      | if strcmp(first,last)
      |     fprintf('%s -- Copyright %s Nexteer',NxtrConf,first)
      | else
      |     fprintf('%s -- %s%s- %s Nexteer',NxtrConf,char(169),first,last)
      | end
  Logical Operator : Logic  Operator=OR  Inputs=3  AllPortsSameDT=off  OutDataTypeStr=boolean
  Logical Operator1 : Logic  Operator=NOT  IconShape=distinctive  AllPortsSameDT=off  OutDataTypeStr=boolean
  PrtclChkENDEF : Outport
  wires:
  Logical Operator/1 -> Logical Operator1/1
  MotCtrlMotCurrAdcVlyDAdcFaild/1 -> Logical Operator/1
  MotCtrlMotCurrAdcVlyEAdcFaild/1 -> Logical Operator/2
  MotCtrlMotCurrAdcVlyFAdcFaild/1 -> Logical Operator/3
  Logical Operator1/1 -> PrtclChkENDEF/1

== system ES200A_CurrMeas/CurrMeas/CurrMeasPer2/CopyRight2 ==

== system ES200A_CurrMeas/CurrMeas/CurrMeasPer2/FltInj_f32 ==
  note: This block requires no modification by FDD author.
      |
      | This block does not actually simulate any fault injection.  It is simply a pass-thru.
      |
      | The Constant port (#2) simply terminates its signal, but we are trying to force the FDD author
      | to properly use the FltInjectionLocType enumeration in FDD model.
  note: EA4.x Fault Injection
  Signal_In : Inport
  Constant : Inport  Port=2
  CopyRight2 : Subsystem  Description=|  mask(Copyright Information){none=on}
      | Copyright info block.                                               
      |                                                                     
      | Place copyright information at the top of every subsystem in design.
      mask prompts: none "No parameters"
      mask help: Place copyright information at the top of every subsystem in design.
      mask Display:
      | NxtrConf = 'Nexteer Confidential';
      | 
      | sys = bdroot; %handle for the current model ("system")
      | first = get_param(sys,'Created');
      | first = first(end-3:end);  %year is last four digits
      | 
      | last = get_param(sys,'LastModifiedDate');
      | if isempty(last)
      |     last = datestr(now,'yyyy');
      | else
      |     last = last(end-3:end);
      | end
      | 
      | if strcmp(first,last)
      |     fprintf('%s -- Copyright %s Nexteer',NxtrConf,first)
      | else
      |     fprintf('%s -- %s%s- %s Nexteer',NxtrConf,char(169),first,last)
      | end
  Terminator : Terminator
  Signal_Out : Outport
  wires:
  Signal_In/1 -> Signal_Out/1
  Constant/1 -> Terminator/1

== system ES200A_CurrMeas/CurrMeas/CurrMeasPer3/Chart1/GetNtc5DQlfrSts ==
  NtcNr : Inport
  f : TriggerPort  TriggerType=function-call
      settings: CopyFcn=Stateflow.SLINSF.SimulinkMan.removeBlockPreDeleteFcn  PreDeleteFcn=Stateflow.SLINSF.SimulinkMan.unsafePredeleteFcn
  CopyRight2 : Subsystem  Description=|  mask(Copyright Information){none=on}
      | Copyright info block.                                               
      |                                                                     
      | Place copyright information at the top of every subsystem in design.
      mask prompts: none "No parameters"
      mask help: Place copyright information at the top of every subsystem in design.
      mask Display:
      | NxtrConf = 'Nexteer Confidential';
      | 
      | sys = bdroot; %handle for the current model ("system")
      | first = get_param(sys,'Created');
      | first = first(end-3:end);  %year is last four digits
      | 
      | last = get_param(sys,'LastModifiedDate');
      | if isempty(last)
      |     last = datestr(now,'yyyy');
      | else
      |     last = last(end-3:end);
      | end
      | 
      | if strcmp(first,last)
      |     fprintf('%s -- Copyright %s Nexteer',NxtrConf,first)
      | else
      |     fprintf('%s -- %s%s- %s Nexteer',NxtrConf,char(169),first,last)
      | end
  GetNtcQlfrSts : Subsystem
  NtcQlfr : Outport
  wires:
  NtcNr/1 -> GetNtcQlfrSts/1(NtcNr)
  GetNtcQlfrSts/1(NtcQlfr) -> NtcQlfr/1

== system ES200A_CurrMeas/CurrMeas/CurrMeasPer3/Chart1/GetNtc6DQlfrSts ==
  NtcNr : Inport
  f : TriggerPort  TriggerType=function-call
      settings: CopyFcn=Stateflow.SLINSF.SimulinkMan.removeBlockPreDeleteFcn  PreDeleteFcn=Stateflow.SLINSF.SimulinkMan.unsafePredeleteFcn
  CopyRight2 : Subsystem  Description=|  mask(Copyright Information){none=on}
      | Copyright info block.                                               
      |                                                                     
      | Place copyright information at the top of every subsystem in design.
      mask prompts: none "No parameters"
      mask help: Place copyright information at the top of every subsystem in design.
      mask Display:
      | NxtrConf = 'Nexteer Confidential';
      | 
      | sys = bdroot; %handle for the current model ("system")
      | first = get_param(sys,'Created');
      | first = first(end-3:end);  %year is last four digits
      | 
      | last = get_param(sys,'LastModifiedDate');
      | if isempty(last)
      |     last = datestr(now,'yyyy');
      | else
      |     last = last(end-3:end);
      | end
      | 
      | if strcmp(first,last)
      |     fprintf('%s -- Copyright %s Nexteer',NxtrConf,first)
      | else
      |     fprintf('%s -- %s%s- %s Nexteer',NxtrConf,char(169),first,last)
      | end
  GetNtcQlfrSts : Subsystem
  NtcQlfr : Outport
  wires:
  NtcNr/1 -> GetNtcQlfrSts/1(NtcNr)
  GetNtcQlfrSts/1(NtcQlfr) -> NtcQlfr/1

== system ES200A_CurrMeas/CurrMeas/CurrMeasPer3/Chart1/RangeChkWIABC ==
  MotCtrlMotCurrAdcVlyA : Inport
  MotCtrlMotCurrAdcVlyB : Inport  Port=2
  MotCtrlMotCurrAdcVlyC : Inport  Port=3
  f : TriggerPort  TriggerType=function-call
      settings: CopyFcn=Stateflow.SLINSF.SimulinkMan.removeBlockPreDeleteFcn  PreDeleteFcn=Stateflow.SLINSF.SimulinkMan.unsafePredeleteFcn
  Constant1 : Constant  Value=CurrMeasMotCurrAdcVlyWrmIninMax
  Constant8 : Constant  Value=CurrMeasMotCurrAdcVlyWrmIninMin
  CopyRight2 : Subsystem  Description=|  mask(Copyright Information){none=on}
      | Copyright info block.                                               
      |                                                                     
      | Place copyright information at the top of every subsystem in design.
      mask prompts: none "No parameters"
      mask help: Place copyright information at the top of every subsystem in design.
      mask Display:
      | NxtrConf = 'Nexteer Confidential';
      | 
      | sys = bdroot; %handle for the current model ("system")
      | first = get_param(sys,'Created');
      | first = first(end-3:end);  %year is last four digits
      | 
      | last = get_param(sys,'LastModifiedDate');
      | if isempty(last)
      |     last = datestr(now,'yyyy');
      | else
      |     last = last(end-3:end);
      | end
      | 
      | if strcmp(first,last)
      |     fprintf('%s -- Copyright %s Nexteer',NxtrConf,first)
      | else
      |     fprintf('%s -- %s%s- %s Nexteer',NxtrConf,char(169),first,last)
      | end
  If Action Subsystem2 : Subsystem  TreatAsAtomicUnit=on
  If Action Subsystem3 : Subsystem  TreatAsAtomicUnit=on
  If1 : If  NumInputs=5  IfExpression=u1>u4 & u2>u4 & u3>u4 & u1<u5 & u2<u5 & u3<u5
  Merge : Merge
  RangeCheckWIABC : Outport
  wires:
  If Action Subsystem3/1(Out1) -> Merge/2
  If Action Subsystem2/1(Out1) -> Merge/1
  MotCtrlMotCurrAdcVlyA/1 -> If1/1
  MotCtrlMotCurrAdcVlyB/1 -> If1/2
  MotCtrlMotCurrAdcVlyC/1 -> If1/3
  Merge/1 -> RangeCheckWIABC/1
  If1/1 -> If Action Subsystem2/Action
  If1/2 -> If Action Subsystem3/Action
  Constant8/1 -> If1/4
  Constant1/1 -> If1/5

== system ES200A_CurrMeas/CurrMeas/CurrMeasPer3/Chart1/RangeChkWIDEF ==
  MotCtrlMotCurrAdcVlyD : Inport
  MotCtrlMotCurrAdcVlyE : Inport  Port=2
  MotCtrlMotCurrAdcVlyF : Inport  Port=3
  f : TriggerPort  TriggerType=function-call
      settings: CopyFcn=Stateflow.SLINSF.SimulinkMan.removeBlockPreDeleteFcn  PreDeleteFcn=Stateflow.SLINSF.SimulinkMan.unsafePredeleteFcn
  Constant1 : Constant  Value=CurrMeasMotCurrAdcVlyWrmIninMax
  Constant8 : Constant  Value=CurrMeasMotCurrAdcVlyWrmIninMin
  CopyRight2 : Subsystem  Description=|  mask(Copyright Information){none=on}
      | Copyright info block.                                               
      |                                                                     
      | Place copyright information at the top of every subsystem in design.
      mask prompts: none "No parameters"
      mask help: Place copyright information at the top of every subsystem in design.
      mask Display:
      | NxtrConf = 'Nexteer Confidential';
      | 
      | sys = bdroot; %handle for the current model ("system")
      | first = get_param(sys,'Created');
      | first = first(end-3:end);  %year is last four digits
      | 
      | last = get_param(sys,'LastModifiedDate');
      | if isempty(last)
      |     last = datestr(now,'yyyy');
      | else
      |     last = last(end-3:end);
      | end
      | 
      | if strcmp(first,last)
      |     fprintf('%s -- Copyright %s Nexteer',NxtrConf,first)
      | else
      |     fprintf('%s -- %s%s- %s Nexteer',NxtrConf,char(169),first,last)
      | end
  If Action Subsystem2 : Subsystem  TreatAsAtomicUnit=on
  If Action Subsystem3 : Subsystem  TreatAsAtomicUnit=on
  If1 : If  NumInputs=5  IfExpression=u1>u4 & u2>u4 & u3>u4 & u1<u5 & u2<u5 & u3<u5
  Merge1 : Merge
  RangeCheckWIDEF : Outport
  wires:
  MotCtrlMotCurrAdcVlyD/1 -> If1/1
  MotCtrlMotCurrAdcVlyE/1 -> If1/2
  MotCtrlMotCurrAdcVlyF/1 -> If1/3
  If1/1 -> If Action Subsystem2/Action
  If1/2 -> If Action Subsystem3/Action
  Merge1/1 -> RangeCheckWIDEF/1
  If Action Subsystem3/1(Out1) -> Merge1/2
  If Action Subsystem2/1(Out1) -> Merge1/1
  Constant8/1 -> If1/4
  Constant1/1 -> If1/5

== system ES200A_CurrMeas/CurrMeas/CurrMeasPer3/Chart1/SetNtc5DSts ==
  NTCNr : Inport
  ParamBit : Inport  Port=2
  NTCSts : Inport  Port=3
  NTCDebStep : Inport  Port=4
  f : TriggerPort  TriggerType=function-call
      settings: CopyFcn=Stateflow.SLINSF.SimulinkMan.removeBlockPreDeleteFcn  PreDeleteFcn=Stateflow.SLINSF.SimulinkMan.unsafePredeleteFcn
  CopyRight2 : Subsystem  Description=|  mask(Copyright Information){none=on}
      | Copyright info block.                                               
      |                                                                     
      | Place copyright information at the top of every subsystem in design.
      mask prompts: none "No parameters"
      mask help: Place copyright information at the top of every subsystem in design.
      mask Display:
      | NxtrConf = 'Nexteer Confidential';
      | 
      | sys = bdroot; %handle for the current model ("system")
      | first = get_param(sys,'Created');
      | first = first(end-3:end);  %year is last four digits
      | 
      | last = get_param(sys,'LastModifiedDate');
      | if isempty(last)
      |     last = datestr(now,'yyyy');
      | else
      |     last = last(end-3:end);
      | end
      | 
      | if strcmp(first,last)
      |     fprintf('%s -- Copyright %s Nexteer',NxtrConf,first)
      | else
      |     fprintf('%s -- %s%s- %s Nexteer',NxtrConf,char(169),first,last)
      | end
  Ground1 : Ground
  SetNtcSts : Subsystem
  MotCurrNtcSet1 : Outport
  wires:
  NTCDebStep/1 -> SetNtcSts/4(DebStep)
  NTCSts/1 -> SetNtcSts/3(NtcSts)
  ParamBit/1 -> SetNtcSts/2(NtcStInfo)
  NTCNr/1 -> SetNtcSts/1(NtcNr)
  Ground1/1 -> MotCurrNtcSet1/1

== system ES200A_CurrMeas/CurrMeas/CurrMeasPer3/Chart1/SetNtc6DSts ==
  NTCNr : Inport
  ParamBit : Inport  Port=2
  NTCSts : Inport  Port=3
  NTCDebStep : Inport  Port=4
  f : TriggerPort  TriggerType=function-call
      settings: CopyFcn=Stateflow.SLINSF.SimulinkMan.removeBlockPreDeleteFcn  PreDeleteFcn=Stateflow.SLINSF.SimulinkMan.unsafePredeleteFcn
  CopyRight2 : Subsystem  Description=|  mask(Copyright Information){none=on}
      | Copyright info block.                                               
      |                                                                     
      | Place copyright information at the top of every subsystem in design.
      mask prompts: none "No parameters"
      mask help: Place copyright information at the top of every subsystem in design.
      mask Display:
      | NxtrConf = 'Nexteer Confidential';
      | 
      | sys = bdroot; %handle for the current model ("system")
      | first = get_param(sys,'Created');
      | first = first(end-3:end);  %year is last four digits
      | 
      | last = get_param(sys,'LastModifiedDate');
      | if isempty(last)
      |     last = datestr(now,'yyyy');
      | else
      |     last = last(end-3:end);
      | end
      | 
      | if strcmp(first,last)
      |     fprintf('%s -- Copyright %s Nexteer',NxtrConf,first)
      | else
      |     fprintf('%s -- %s%s- %s Nexteer',NxtrConf,char(169),first,last)
      | end
  Ground1 : Ground
  SetNtcSts : Subsystem
  MotCurrNtcSet2 : Outport
  wires:
  NTCDebStep/1 -> SetNtcSts/4(DebStep)
  NTCSts/1 -> SetNtcSts/3(NtcSts)
  ParamBit/1 -> SetNtcSts/2(NtcStInfo)
  NTCNr/1 -> SetNtcSts/1(NtcNr)
  Ground1/1 -> MotCurrNtcSet2/1

== system ES200A_CurrMeas/CurrMeas/CurrMeasPer3/CopyRight2 ==

== system ES200A_CurrMeas/CurrMeas/FltInj_f32/CopyRight2 ==
